simulink model "VehicleSimulation"  (R2018b)
settings: Solver=FixedStepAuto  StartTime=0.0  StopTime=Tsim  FixedStep=Ts  RelTol=1e-6
values from neighbouring files (symbols this model uses):
  Ts = 0.01    [modelFitEDMD.m]
  Tsim = (Nsim-1)*Ts    [simulationEDMD.m]
  x0 = xLowLim + rand(nx,Ntraj).*(xUppLim - xLowLim)    [errorAnalysis.m]    (also in simulationEDMD.m = [32.5698; -9.1526; 2.5326])
libraries: simulink x1, simulink_extras x1
settings Model: Creator=Marko  LastModifiedBy=Marko

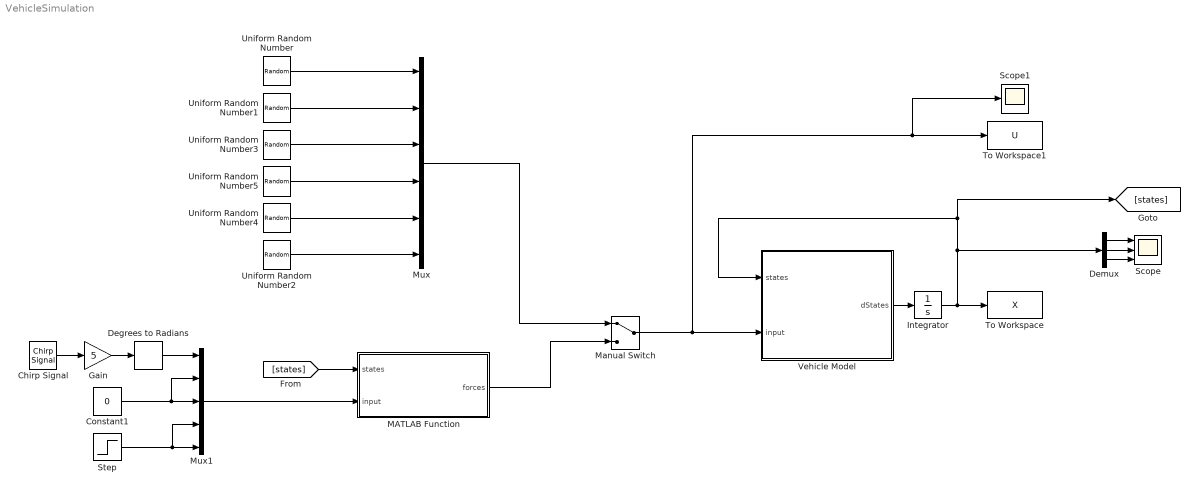
== system VehicleSimulation ==
  Chirp Signal : simulink/Sources/Chirp Signal  f1=0.1  T=Tsim  f2=10
  Constant1 : Constant  Value=0
  Degrees to Radians : simulink_extras/Transformations/Degrees to Radians
  Demux : Demux  Outputs=3
  Gain : Gain  Gain=5
  Integrator : Integrator  InitialCondition=x0
  MATLAB Function : MATLAB Function  TreatAsAtomicUnit=on
  Manual Switch : ManualSwitch
  Mux : Mux  Inputs=6
  Mux1 : Mux  Inputs=5
  Scope : Scope  NumInputPorts=3
  Scope1 : Scope
  Step : Step  Time=3  Before=0.15  After=0  SampleTime=0
  To Workspace : ToWorkspace  VariableName=X  SampleTime=Ts
  To Workspace1 : ToWorkspace  VariableName=U  SampleTime=Ts
  Uniform Random Number : UniformRandomNumber  Minimum=-10000  Maximum=10000  Seed=5  SampleTime=Ts
  Uniform Random Number1 : UniformRandomNumber  Minimum=-10000  Maximum=10000  Seed=256  SampleTime=Ts
  Uniform Random Number2 : UniformRandomNumber  Minimum=-10000  Maximum=10000  Seed=156  SampleTime=Ts
  Uniform Random Number3 : UniformRandomNumber  Minimum=-10000  Maximum=10000  Seed=210  SampleTime=Ts
  Uniform Random Number4 : UniformRandomNumber  Minimum=-10000  Maximum=10000  Seed=24546354  SampleTime=Ts
  Uniform Random Number5 : UniformRandomNumber  Minimum=-10000  Maximum=10000  Seed=555  SampleTime=Ts
  Vehicle Model : MATLAB Function  TreatAsAtomicUnit=on
  wires:
  Vehicle Model/1(dStates) -> Integrator/1
  Integrator/1 -> To Workspace/1, Demux/1, [states], Vehicle Model/1(states)
  Demux/1 -> Scope/1
  Demux/2 -> Scope/2
  Demux/3 -> Scope/3
  Mux/1 -> Manual Switch/1
  Manual Switch/1 -> Scope1/1, To Workspace1/1, Vehicle Model/2(input)
  Uniform Random Number/1 -> Mux/1
  Uniform Random Number1/1 -> Mux/2
  Uniform Random Number4/1 -> Mux/5
  Uniform Random Number2/1 -> Mux/6
  Uniform Random Number3/1 -> Mux/3
  Uniform Random Number5/1 -> Mux/4
  Gain/1 -> Degrees to Radians/1
  Degrees to Radians/1 -> Mux1/1
  Mux1/1 -> MATLAB Function/2(input)
  [states] -> MATLAB Function/1(states)
  Constant1/1 -> Mux1/2, Mux1/3
  Chirp Signal/1 -> Gain/1
  Step/1 -> Mux1/4, Mux1/5
  MATLAB Function/1(forces) -> Manual Switch/2

== matlab function VehicleSimulation/MATLAB Function ==
  data: states input; forces output; input input
function forces = ForceGenerator(states, input)
% VEHICLE MODEL 
%   The function accepts current system states and inputs, and calculates 
%   state derivatives.

% States and input definition

vx = states(1);
vy = states(2);
omega = states(3);

deltaF = input(1);
sfl = input(2);
sfr = input(3);
srl = input(4);
srr = input(5);

% Initialize vehicle parameters
vehicle = LoadVehicleParameters();

lf = vehicle.lf;
lr = vehicle.lr;
w = vehicle.w;
m = vehicle.m;
Jz = vehicle.Jz;

% Air drag parameters
cw = vehicle.cw;
rho = vehicle.rho;
Aw = vehicle.Aw;

% VEHICLE VELOCITIES

% Longitudinal velocities
vxfl = vx - w*omega;
vxfr = vx + w*omega;
vxrl = vx - w*omega;
vxrr = vx + w*omega;
% Lateral velocities
vyfl = vy + lf*omega;
vyfr = vy + lf*omega;
vyrl = vy - lr*omega;
vyrr = vy - lr*omega;

% TYRE VELOCITIES

% Longitudinal velocities
vlfl = vxfl*cos(deltaF) + vyfl*sin(deltaF);
vlfr = vxfr*cos(deltaF) + vyfr*sin(deltaF);
vlrl = vxrl;
vlrr = vxrr;

% Cornering velocities
vcfl = -vxfl*sin(deltaF) + vyfl*cos(deltaF);
vcfr = -vxfr*sin(deltaF) + vyfr*cos(deltaF);
vcrl = vyrl;
vcrr = vyrr;

% TYRE SLIP ANGLES
alpha_fl = atan2(vcfl,vlfl);
alpha_fr = atan2(vcfr,vlfr);
alpha_rl = atan2(vcrl,vlrl);
alpha_rr = atan2(vcrr,vlrr);

% TYRE FORCES
Cx = vehicle.Cx;
Cy = vehicle.Cy;

% Longitudinal forces
Flfl = Cx*sfl;
Flfr = Cx*sfr;
Flrl = Cx*srl;
Flrr = Cx*srr;

% Conrnering forces
Fcfl = -Cy*alpha_fl;
Fcfr = -Cy*alpha_fr;
Fcrl = -Cy*alpha_rl;
Fcrr = -Cy*alpha_rr;

% AXLE FORCES

% Longitudinal forces
Fxfl = Flfl*cos(deltaF) - Fcfl*sin(deltaF);
Fxfr = Flfr*cos(deltaF) - Fcfr*sin(deltaF);
Fxrl = Flrl;
Fxrr = Flrr;

% Lateral forces
Fyfl = Flfl*sin(deltaF) + Fcfl*cos(deltaF);
Fyfr = Flfr*sin(deltaF) + Fcfr*cos(deltaF);
Fyrl = Fcrl;
Fyrr = Fcrr;

forces = [Fxfl; Fyfl; Fxfr; Fyfr; Fxrl; Fxrr];

end

== matlab function VehicleSimulation/Vehicle Model ==
  data: states input; dStates output; input input
function dStates = VehicleModel(states, input)
% VEHICLE MODEL 
%   The function accepts current system states and inputs, and calculates 
%   state derivatives.

% State definition
vx = states(1);
vy = states(2);
omega = states(3);

% Input definition
Fxfl = input(1);
Fyfl = input(2);
Fxfr = input(3);
Fyfr = input(4);
Fxrl = input(5);
Fxrr = input(6);

% Initialize vehicle parameters
vehicle = LoadVehicleParameters();

% Vehicle parameters
lf = vehicle.lf;
lr = vehicle.lr;
w = vehicle.w;
m = vehicle.m;
Jz = vehicle.Jz;

% Air drag parameters
cw = vehicle.cw;
rho = vehicle.rho;
Aw = vehicle.Aw;

% VEHICLE VELOCITIES

% Lateral velocities
vyrl = vy - lr*omega;
vyrr = vy - lr*omega;
% Longitudinal velocities
vxrl = vx - w*omega;
vxrr = vx + w*omega;

% TIRE VELOCITIES

% Cornering velocities
vcrl = vyrl;
vcrr = vyrr;

% Longitudinal velocities
vlrl = vxrl;
vlrr = vxrr;

% TIRE SLIP ANGLES

alpha_rl = atan2(vcrl,vlrl);
alpha_rr = atan2(vcrr,vlrr);

% TIRE FORCES
Cy = vehicle.Cy;

% Conrnering forces
Fcrl = -Cy*alpha_rl;
Fcrr = -Cy*alpha_rr;

% AXLE FORCES

% Lateral forces
Fyrl = Fcrl;
Fyrr = Fcrr;

% VEHICLE DYNAMICS MODEL

dvx = vy*omega + 1/m *(-0.5*cw*rho*Aw*sqrt(vx^2+vy^2)*vx + Fxfl + Fxfr + Fxrl + Fxrr);
dvy = -vx*omega + 1/m *(-0.5*cw*rho*Aw*sqrt(vx^2+vy^2)*vy + Fyfl + Fyfr + Fyrl + Fyrr);
dOmega = lf/Jz*(Fyfl + Fyfr) - lr/Jz*(Fyrl + Fyrr) + w/Jz*(-Fxfl + Fxfr -Fxrl + Fxrr);

dStates = [dvx; dvy; dOmega];
end
